simulink model "AMP_simulink"  (R2024b)
settings: Solver=VariableStepAuto  StartTime=0.0  StopTime=5  RelTol=1e-3
InitFcn:
  | R1=5e6;
  | R2=R1;
  | R3=R2;
  | C1=100e-9;
  | C2=C1;
  | V=5;

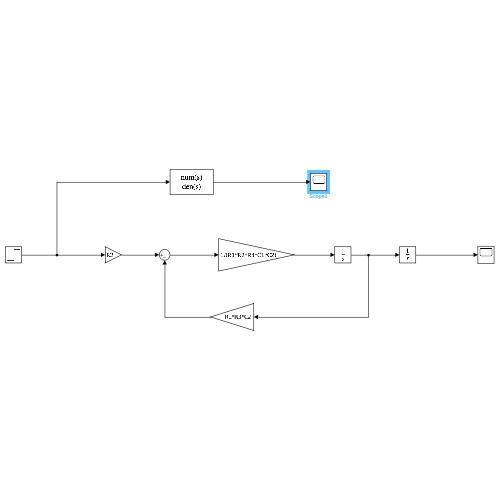
[thumbnail: Simulink's stored preview of the top-level diagram]
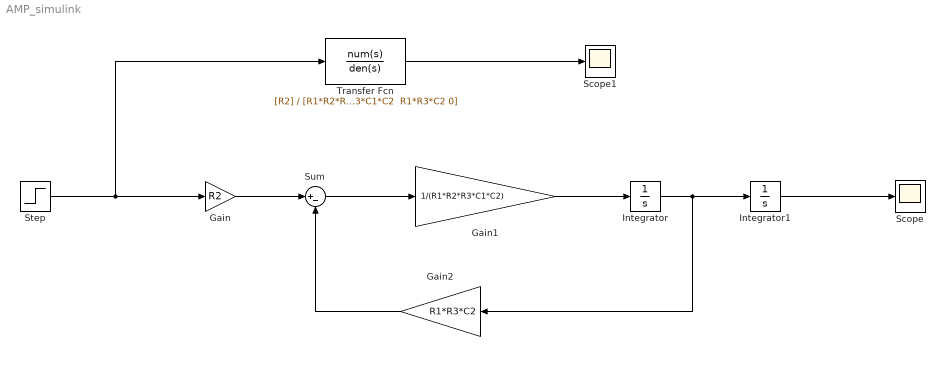
== system AMP_simulink ==
  Gain : Gain  Gain=R2
  Gain1 : Gain  Gain=1/(R1*R2*R3*C1*C2)
  Gain2 : Gain  Gain=R1*R3*C2
  Integrator : Integrator
  Integrator1 : Integrator
  Scope : Scope
  Scope1 : Scope
  Step : Step  Time=0  After=5  SampleTime=0
  Sum : Sum  Inputs=|+-
  Transfer Fcn : TransferFcn  Numerator=[R2]  Denominator="[R1*R2*R3*C1*C2  R1*R3*C2 0]"
  wires:
  Gain/1 -> Sum/1
  Step/1 -> Transfer Fcn/1, Gain/1
  Sum/1 -> Gain1/1
  Gain2/1 -> Sum/2
  Integrator/1 -> Gain2/1, Integrator1/1
  Gain1/1 -> Integrator/1
  Integrator1/1 -> Scope/1
  Transfer Fcn/1 -> Scope1/1
